simulink model "wind_model"  (R2019a)
settings: Solver=FixedStepAuto  StartTime=0.0  StopTime=300  FixedStep=0.1  RelTol=1e-3
undefined symbols (not defined in the file or in its folder): useWindM
libraries: simulink x3
settings Model: Creator=Wai-Yen Chan  LastModifiedBy=den

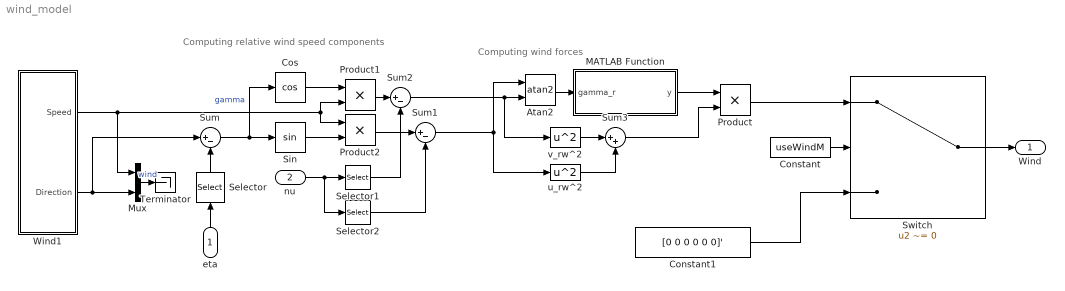
== system wind_model ==
  note: Computing relative wind speed components
  note: Computing wind forces
  eta : Inport  PortDimensions=3
  nu : Inport  Port=2  PortDimensions=3
  Atan2 : Trigonometry  Operator=atan2
  Constant : Constant  Value=useWindM
  Constant1 : Constant  Value=[0 0 0 0 0 0]'
  Cos : Trigonometry  Operator=cos
  MATLAB Function : MATLAB Function  TreatAsAtomicUnit=on
  Mux : Mux  Inputs=2
  Product : Product
  Product1 : Product
  Product2 : Product
  Selector : Selector  InputPortWidth=3  IndexOptions=Index vector (dialog)  Indices=[3]  OutputSizes=1
  Selector1 : Selector  InputPortWidth=3  IndexOptions=Index vector (dialog)  Indices=[1]  OutputSizes=1
  Selector2 : Selector  InputPortWidth=3  IndexOptions=Index vector (dialog)  Indices=[2]  OutputSizes=1
  Sin : Trigonometry
  Sum : Sum  Inputs=|+-
  Sum1 : Sum  Inputs=|+-
  Sum2 : Sum  Inputs=|+-
  Sum3 : Sum  Inputs=|++
  Switch : Switch  Criteria=u2 ~= 0
  Terminator : Terminator
  Wind1 : Subsystem  mask{u_mean_10=10, height=3, kappa=0.0026, dir_mean=pi, dir_time_constant=10, dir_lim=pi/36, usv_time_constant=100, usv_lim=1, np_usv=5, np_dir=0.05, N=100}
      mask DialogControl Control6 Prompt: Mean wind speed at 10m height [m/s]
      mask DialogControl Control10 Prompt: Height above water surface [m]
      mask DialogControl Control11 Prompt: Sea surface drag coefficient
      mask DialogControl Control7 Prompt: Mean wind direction [rad]
      mask DialogControl Control4 Prompt: Direction Time Constant [s]
      mask DialogControl Control5 Prompt: Direction Limit [rad]
      mask DialogControl Control3 Prompt: Slowly varying Time Constant [s]
      mask DialogControl Control2 Prompt: Slowly varying Limit [m/s]
      mask DialogControl Control8 Prompt: Usv noise power
      mask DialogControl Control9 Prompt: Direction noise power
      mask DialogControl Control12 Prompt: Frequency component count
  u_rw^2 : Math  Operator=square  SaturateOnIntegerOverflow=on
  v_rw^2 : Math  Operator=square  SaturateOnIntegerOverflow=on
  Wind : Outport  PortDimensions=6
  wires:
  MATLAB Function/1(y) -> Product/1
  Sum/1 -> Cos/1, Sin/1  "gamma"
  Wind1/2(Direction) -> Mux/2, Sum/1
  nu/1 -> Selector2/1, Selector1/1
  Selector1/1 -> Sum2/2
  Cos/1 -> Product1/1
  Wind1/1(Speed) -> Product1/2, Product2/1, Mux/1
  Sin/1 -> Product2/2
  Product1/1 -> Sum2/1
  Product2/1 -> Sum1/1
  Selector2/1 -> Sum1/2
  u_rw^2/1 -> Sum3/2
  v_rw^2/1 -> Sum3/1
  Sum3/1 -> Product/2
  Sum2/1 -> Atan2/2, v_rw^2/1
  Sum1/1 -> u_rw^2/1, Atan2/1
  Atan2/1 -> MATLAB Function/1(gamma_r)
  eta/1 -> Selector/1
  Selector/1 -> Sum/2
  Product/1 -> Switch/1
  Switch/1 -> Wind/1
  Constant/1 -> Switch/2
  Constant1/1 -> Switch/3
  Mux/1 -> Terminator/1  "wind"

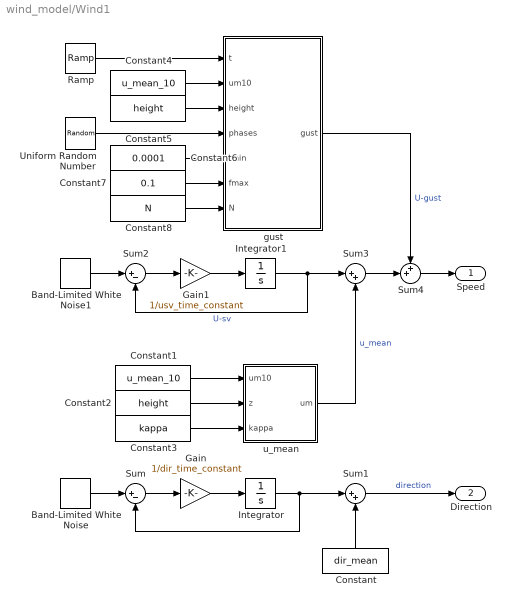
== system wind_model/Wind1 ==
  Band-Limited White Noise : simulink/Sources/Band-Limited White Noise  Cov=np_dir  Ts=0.1  seed=[11311]
  Band-Limited White Noise1 : simulink/Sources/Band-Limited White Noise  Cov=[np_usv]  Ts=0.1  seed=[12112]
  Constant : Constant  Value=dir_mean
  Constant1 : Constant  Value=u_mean_10
  Constant2 : Constant  Value=height
  Constant3 : Constant  Value=kappa
  Constant4 : Constant  Value=u_mean_10
  Constant5 : Constant  Value=height
  Constant6 : Constant  Value=0.0001
  Constant7 : Constant  Value=0.1
  Constant8 : Constant  Value=N
  Gain : Gain  Gain=1/dir_time_constant
  Gain1 : Gain  Gain=1/usv_time_constant
  Integrator : Integrator  LimitOutput=on  UpperSaturationLimit=dir_lim  LowerSaturationLimit=-dir_lim
  Integrator1 : Integrator  LimitOutput=on  UpperSaturationLimit=usv_lim  LowerSaturationLimit=-usv_lim
  Ramp : simulink/Sources/Ramp  slope=1  start=0  InitialOutput=0
  Sum : Sum  Inputs=|+-
  Sum1 : Sum  Inputs=|++
  Sum2 : Sum  Inputs=|+-
  Sum3 : Sum  Inputs=|++
  Sum4 : Sum  Inputs=++|
  Uniform Random Number : UniformRandomNumber  Minimum=-pi*ones(N,1)  Maximum=pi*ones(N,1)  Seed=double(uint32(121010101*rand(N,1)))  SampleTime=1e5
  gust : MATLAB Function  TreatAsAtomicUnit=on
  u_mean : MATLAB Function  TreatAsAtomicUnit=on
  Speed : Outport
  Direction : Outport  Port=2
  wires:
  Integrator/1 -> Sum1/1, Sum/2
  Band-Limited White Noise/1 -> Sum/1
  Sum1/1 -> Direction/1  "direction"
  Constant/1 -> Sum1/2
  Sum/1 -> Gain/1
  Integrator1/1 -> Sum3/1, Sum2/2  "U-sv"
  Constant1/1 -> u_mean/1(um10)
  Band-Limited White Noise1/1 -> Sum2/1
  Sum2/1 -> Gain1/1
  Sum4/1 -> Speed/1
  gust/1(gust) -> Sum4/1  "U-gust"
  u_mean/1(um) -> Sum3/2  "u_mean"
  Constant2/1 -> u_mean/2(z)
  Constant3/1 -> u_mean/3(kappa)
  Ramp/1 -> gust/1(t)
  Gain/1 -> Integrator/1
  Gain1/1 -> Integrator1/1
  Sum3/1 -> Sum4/2
  Constant6/1 -> gust/5(fmin)
  Constant7/1 -> gust/6(fmax)
  Constant8/1 -> gust/7(N)
  Constant4/1 -> gust/2(um10)
  Constant5/1 -> gust/3(height)
  Uniform Random Number/1 -> gust/4(phases)

== matlab function wind_model/Wind1/gust ==
  settings: updateMethod=DISCRETE
  data: t input; um10 input [1..1000]; gust output; height input; phases input [1..1000]; fmin input; fmax input; N input
function gust  = fcn(t, um10, height, phases, fmin, fmax, N)

% linearly spaced components
freqs = linspace(fmin,fmax,N)';
df = freqs(2) - freqs(1);

x = zeros(N,1);

% Norsok spectrum
n = 0.468;
x = 172*freqs*(height/10)^(2/3) * (um10/10)^(-3/4);
x = x.^n;
x = (1+x).^(5/(3*n));
Sf = (320*(um10/10)^2*(height/10)^0.45)./x;

% wind component amplitudes
% amps = zeros(1, N);
% for i = 1:N
%     amps(i) = sqrt(2*Sf(i)*delta_freqs(i));
% end
amps = sqrt(2*Sf.*df);

% wind gust magnitude at this time
% gust = 0;
% for i = 1:N
%     gust = gust + amps(i)*sin(2*pi*freqs(i)*t + 2*pi*rand(1));
%     % gust = gust + amps(i)*sin(2*pi*freqs(i)*t + phases(i));
% end

gust = (amps')*(sin(2*pi*freqs*t + phases));
% gust = (sin(2*pi*freqs*t + phases));

== matlab function wind_model/Wind1/u_mean ==
  data: um10 input; um output; z input; kappa input
function um = fcn(um10, z, kappa)
um = 0;
z0 = 10*exp(-2/(5*sqrt(kappa)));
um = um10*5*sqrt(kappa)*log(z/z0)/2;

== matlab function wind_model/MATLAB Function ==
  data: gamma_r input; y output
function y = fcn(gamma_r)

coder.extrinsic('round')

CN_data = [
  0  248.3700 0 0 0 -2355.232759 0
 10  265.1900 61.332 0 275.994 -2514.732759 551.1
 20  224.1300 136.22 0 612.99 -2125.37069 661.56
 30  149.0300 238.76 0 1074.42 -1413.215517 451.37
 40  134.3600 319.42 0 1437.39 -1274.103448 212.51
 50   96.8000 380.5 0 1712.25 -917.9310345 -23.578
 60   41.3640 396.1 0 1782.45 -392.2448276 1168.3
 70   16.4770 372.96 0 1678.32 -156.2474138 2376.3
 80    0.30412 376.5 0 1694.25 -2.883896552 3511.9
 90   -3.7230 390.01 0 1755.045 35.30431034 4610.4
100  -24.8790 386.63 0 1739.835 235.9215517 4769.5
110  -61.2810 393.76 0 1771.92 581.112931 5921.9
120 -108.5000 408.66 0 1838.97 1028.87931 6542.8
130 -169.3500 393.26 0 1769.67 1605.905172 6805.2
140 -206.6300 276.93 0 1246.185 1959.422414 6751.5
150 -201.9900 200.64 0 902.88 1915.422414 6190.1
160 -196.5100 124.71 0 561.195 1863.456897 3758.8
170 -181.5300 56.27 0 253.215 1721.405172 1905.6
180 -208.2200 0 0 0 1974.5 0
190 -181.5300 -56.27 0 -253.215 1721.405172 -1905.6
200 -196.5100 -124.71 0 -561.195 1863.456897 -3758.8
210 -201.9900 -200.64 0 -902.88 1915.422414 -6190.1
220 -206.6300 -276.93 0 -1246.185 1959.422414 -6751.5
230 -169.3500 -393.26 0 -1769.67 1605.905172 -6805.2
240 -108.5000 -408.66 0 -1838.97 1028.87931 -6542.8
250  -61.2810 -393.76 0 -1771.92 581.112931 -5921.9
260  -24.8790 -386.63 0 -1739.835 235.9215517 -4769.5
270  -3.72300 -390.01 0 -1755.045 35.30431034 -4610.4
280   0.30412 -376.5 0 -1694.25 -2.883896552 -3511.9
290  16.47700 -372.96 0 -1678.32 -156.2474138 -2376.3
300  41.36400 -396.1 0 -1782.45 -392.2448276 -1168.3
310  96.80000 -380.5 0 -1712.25 -917.9310345 23.578
320  134.3600 -319.42 0 -1437.39 -1274.103448 -212.51
330  149.0300 -238.76 0 -1074.42 -1413.215517 -451.37
340  224.1300 -136.22 0 -612.99 -2125.37069 -661.56
350  265.1900 -61.332 0 -275.994 -2514.732759 -551.1
360  248.3700 0 0 0 -2355.232759 0];


gamma_r = rad2deg(mod(gamma_r, 2*pi));

% Linear interpolation between points
Cx = interp1(CN_data(:, 1), CN_data(:, 2), gamma_r);
Cy = interp1(CN_data(:, 1), CN_data(:, 3), gamma_r);
Cz = 0;
Ctheta = interp1(CN_data(:, 1), CN_data(:, 5), gamma_r);
Cphi = interp1(CN_data(:, 1), CN_data(:, 6), gamma_r);
Cpsi = interp1(CN_data(:, 1), CN_data(:, 7), gamma_r);

y = [Cx Cy Cz Ctheta Cphi Cpsi]';
